simulink library "mylib"  (Simulink 7.3)
settings: Solver=ode45  StartTime=0.0  StopTime=10.0  RelTol=1e-3
settings Model: Creator=Krisada  LastModifiedBy=Krisada

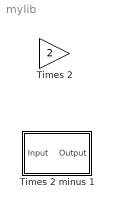
== system mylib ==
  Times 2 : Gain  Gain=2  ParameterDataType=fixdt(1, 16)  ParameterScaling=2^0  OutDataType=fixdt(1, 16)  OutScaling=2^0
  Times 2 minus 1 : Subsystem

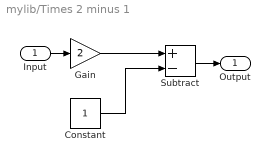
== system mylib/Times 2 minus 1 ==
  Input : Inport
  Constant : Constant  OutDataType=fixdt(1, 16)  OutScaling=2^0
  Gain : Gain  Gain=2  ParameterDataType=fixdt(1, 16)  ParameterScaling=2^0  OutDataType=fixdt(1, 16)  OutScaling=2^0
  Subtract : Sum  Inputs=+-  OutDataType=fixdt(1, 16)  OutScaling=2^-10
  Output : Outport
  wires:
  Gain/1 -> Subtract/1
  Constant/1 -> Subtract/2
  Input/1 -> Gain/1
  Subtract/1 -> Output/1
